simulink model "lqrpilot"  (Simulink 4.00)
settings: Solver=ode45  StartTime=0.0  StopTime=60  RelTol=1e-3
PreLoadFcn:
  | load lqrpilot
values from neighbouring files (symbols this model uses):
  A15 = A + [zeros(8,4) A_nl]    [lqrdes.m]
  B = [.00729  0 ... (first row only)    [jetdemo.m]    (also in kalmdemo.m = [-0.3832; lqrdes.m = [ 20.3929   -0.4694   -0.2392   -0.7126)
  K_lqr = lqry(dc_aug,diag([1 20]),0.01)    [dcdemo.m]    (also in lqrdes.m = lqr(A_aug,B_aug,Q,R))
libraries: simulink3 x1
settings Model: Creator=pascal  LastModifiedBy=eyarrow  AlgebraicLoopMsg=none  BlockReductionOpt=off

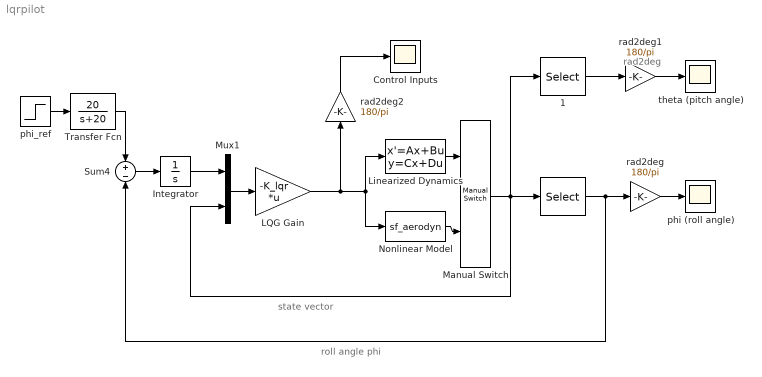
== system lqrpilot ==
  note: state vector
  note: roll angle phi
  note: rad2deg
  " " : Selector  InputType=Vector  ElementSrc=Internal  Elements=8  RowSrc=Internal  Rows=1  ColumnSrc=Internal  Columns=1  InputPortWidth=8
  " 1" : Selector  InputType=Vector  ElementSrc=Internal  Elements=7  RowSrc=Internal  Rows=1  ColumnSrc=Internal  Columns=1  InputPortWidth=8
  Control Inputs : Scope
      settings: TimeRange=60  YMin=-30  YMax=15  SaveToWorkspace=off  SaveName=ScopeData2  MaxDataPoints=5000
  Integrator : Integrator  ExternalReset=none  InitialConditionSource=internal  InitialCondition=0  LimitOutput=off  UpperSaturationLimit=inf  LowerSaturationLimit=-inf  ShowSaturationPort=off  ShowStatePort=off  AbsoluteTolerance=auto
  LQG Gain : Gain  Gain=-K_lqr  Multiplication=Matrix(K*u)  SaturateOnIntegerOverflow=on
  Linearized Dynamics : StateSpace  A=A15  B=B  C=eye(8)  D=zeros(8,4)  X0=0  Realization=auto  AbsoluteTolerance=auto
  Manual Switch : simulink3/Nonlinear/Manual Switch  sw=0  action=0
  Mux1 : Mux  Inputs=2
  Nonlinear Model : S-Function  FunctionName=sf_aerodyn  PortCounts=[]  SFunctionModules=''
  Sum4 : Sum  Inputs=+-  SaturateOnIntegerOverflow=on
  Transfer Fcn : TransferFcn  Numerator=20  Denominator=[1 20]  Realization=auto  AbsoluteTolerance=auto
  phi (roll angle) : Scope
      settings: TimeRange=60  YMin=-20  YMax=60  SaveToWorkspace=off  SaveName=ScopeData  MaxDataPoints=5000
  phi_ref : Step  Time=0  Before=0  After=pi/3  SampleTime=0
  rad2deg : Gain  Gain=180/pi  Multiplication=Element-wise(K.*u)  SaturateOnIntegerOverflow=on
  rad2deg1 : Gain  Gain=180/pi  Multiplication=Element-wise(K.*u)  SaturateOnIntegerOverflow=on
  rad2deg2 : Gain  Orientation=up  Gain=180/pi  Multiplication=Element-wise(K.*u)  SaturateOnIntegerOverflow=on
  theta (pitch angle) : Scope
      settings: TimeRange=60  YMin=-7.5  YMax=10  SaveToWorkspace=off  MaxDataPoints=5000
  wires:
  phi_ref/1 -> Transfer Fcn/1
  Sum4/1 -> Integrator/1
  Mux1/1 -> LQG Gain/1
  Integrator/1 -> Mux1/1
  Transfer Fcn/1 -> Sum4/1
  LQG Gain/1 -> Linearized Dynamics/1, Nonlinear Model/1, rad2deg2/1
  Linearized Dynamics/1 -> Manual Switch/1
  Nonlinear Model/1 -> Manual Switch/2
  rad2deg/1 -> phi (roll angle)/1
  " 1"/1 -> rad2deg1/1
  rad2deg1/1 -> theta (pitch angle)/1
  rad2deg2/1 -> Control Inputs/1
  Manual Switch/1 -> " "/1, " 1"/1, Mux1/2
  " "/1 -> rad2deg/1, Sum4/2
